simulink model "ANNC_Outer_loop_Int_Act"  (R2021b)
settings: Solver=ode4  StartTime=0.0  StopTime=35  FixedStep=1e-3  RelTol=1e-3
settings Model: Creator=hellb  LastModifiedBy=Ivan Lopez
settings SolverCC: AlgebraicLoopSolver=TrustRegion
settings DataIOCC: ReturnWorkspaceOutputs=off
settings DebuggingCC: SFMachineParentedDataDiag=warning  UnderSpecifiedDimensionMsg=warning  ArithmeticOperatorsInVariantConditions=warning
settings SFSimCC: SimUseLocalCustomCode=off  CustomCodeUndefinedFunction=UseInterfaceOnly
settings RTWCC: RTWUseLocalCustomCode=off

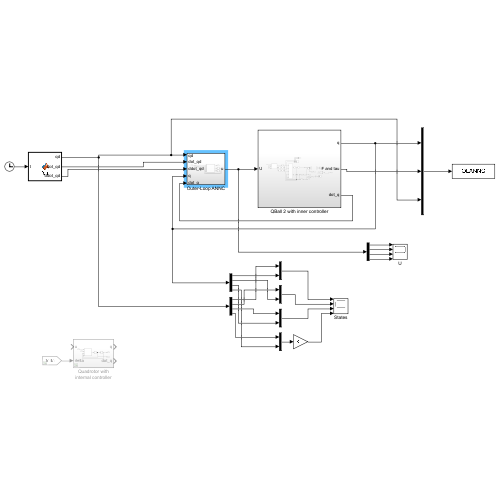
[thumbnail: Simulink's stored preview of the top-level diagram]
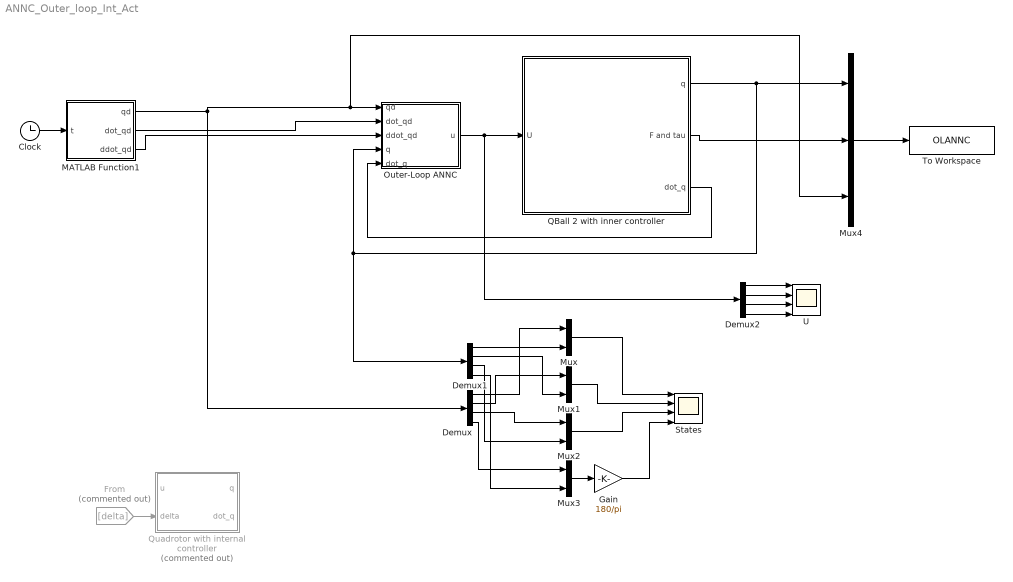
== system ANNC_Outer_loop_Int_Act ==
  Clock : Clock
  Demux : Demux
  Demux1 : Demux
  Demux2 : Demux
  From : From  Commented=on  GotoTag=delta  TagVisibility=global
  Gain : Gain  Gain=180/pi
  MATLAB Function1 : MATLAB Function  TreatAsAtomicUnit=on
  Mux{,1..3} (4 alike) : Mux  Inputs=2
  Mux4 : Mux  Inputs=3
  Outer-Loop ANNC : Subsystem
  QBall 2 with inner controller : Subsystem
  Quadrotor with internal controller : Subsystem  Commented=on
  States : Scope  NumInputPorts=4
  To Workspace : ToWorkspace  VariableName=OLANNC  SaveFormat=Structure With Time  SampleTime=-1
  U : Scope  NumInputPorts=4
  wires:
  Clock/1 -> MATLAB Function1/1(t)
  MATLAB Function1/1(qd) -> Mux4/3, Outer-Loop ANNC/1(qd), Demux/1
  Demux/1 -> Mux/1
  Demux1/1 -> Mux/2
  Demux/2 -> Mux1/1
  Demux1/2 -> Mux1/2
  Demux/3 -> Mux2/1
  Demux1/3 -> Mux2/2
  Demux/4 -> Mux3/1
  Demux1/4 -> Mux3/2
  Mux/1 -> States/1
  Mux1/1 -> States/2
  Mux2/1 -> States/3
  Mux3/1 -> Gain/1
  Gain/1 -> States/4
  From/1 -> Quadrotor with internal controller/2(delta)
  MATLAB Function1/2(dot_qd) -> Outer-Loop ANNC/2(dot_qd)
  MATLAB Function1/3(ddot_qd) -> Outer-Loop ANNC/3(ddot_qd)
  Mux4/1 -> To Workspace/1
  Outer-Loop ANNC/1(u) -> Demux2/1, QBall 2 with inner controller/1(U)
  QBall 2 with inner controller/1(q) -> Outer-Loop ANNC/4(q), Demux1/1, Mux4/1
  QBall 2 with inner controller/3(dot_q) -> Outer-Loop ANNC/5(dot_q)
  Demux2/1 -> U/1
  Demux2/2 -> U/2
  Demux2/3 -> U/3
  Demux2/4 -> U/4
  QBall 2 with inner controller/2(F and tau) -> Mux4/2

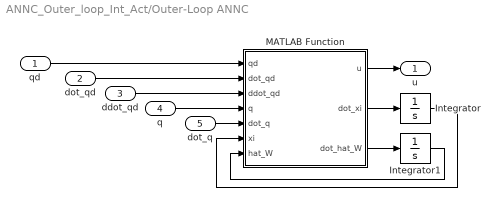
== system ANNC_Outer_loop_Int_Act/Outer-Loop ANNC ==
  qd : Inport
  dot_qd : Inport  Port=2
  ddot_qd : Inport  Port=3
  q : Inport  Port=4
  dot_q : Inport  Port=5
  Integrator : Integrator  InitialCondition=[0;0;0;0]
  Integrator1 : Integrator  InitialCondition=zeros(10,4)
  MATLAB Function : MATLAB Function  TreatAsAtomicUnit=on
  u : Outport  VectorParamsAs1DForOutWhenUnconnected=off
  wires:
  dot_q/1 -> MATLAB Function/5(dot_q)
  q/1 -> MATLAB Function/4(q)
  MATLAB Function/2(dot_xi) -> Integrator/1
  ddot_qd/1 -> MATLAB Function/3(ddot_qd)
  MATLAB Function/1(u) -> u/1
  Integrator1/1 -> MATLAB Function/7(hat_W)
  Integrator/1 -> MATLAB Function/6(xi)
  MATLAB Function/3(dot_hat_W) -> Integrator1/1
  dot_qd/1 -> MATLAB Function/2(dot_qd)
  qd/1 -> MATLAB Function/1(qd)

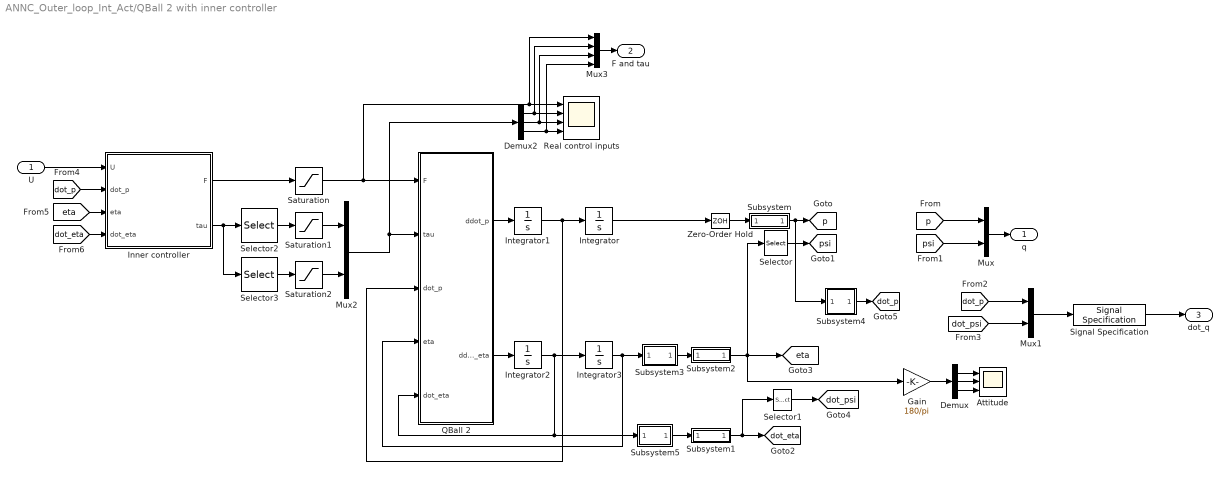
== system ANNC_Outer_loop_Int_Act/QBall 2 with inner controller ==
  U : Inport
  Attitude : Scope  NumInputPorts=3
  Demux : Demux  Outputs=3
  Demux2 : Demux  Outputs=3
  Gain : Gain  Gain=180/pi
  Inner controller : MATLAB Function  TreatAsAtomicUnit=on
  Integrator : Integrator  InitialCondition=[0;0;0.3]  LimitOutput=on  UpperSaturationLimit=[inf;inf;inf]  LowerSaturationLimit=[-inf;-inf;0.3]
  Integrator1 : Integrator  InitialCondition=[0;0;0]
  Integrator2 : Integrator  InitialCondition=[0;0;0]
  Integrator3 : Integrator  InitialCondition=[0;0;0]  LimitOutput=on  UpperSaturationLimit=[pi/2; pi/2; inf]  LowerSaturationLimit=[-pi/2; -pi/2; -inf]
  Mux : Mux  Inputs=2
  Mux1 : Mux  Inputs=2
  Mux2 : Mux  Inputs=2
  Mux3 : Mux
  QBall 2 : MATLAB Function  TreatAsAtomicUnit=on
  Real control inputs : Scope  NumInputPorts=4
  Saturation : Saturate  UpperLimit=8.6*4  LowerLimit=0
  Saturation1 : Saturate  UpperLimit=0.7  LowerLimit=-0.7
  Saturation2 : Saturate  UpperLimit=0.43  LowerLimit=-0.43
  Selector : Selector  InputPortWidth=3  IndexOptions=Index vector (dialog)  Indices=[3]  OutputSizes=1
  Selector1 : Selector  InputPortWidth=3  IndexOptions=Index vector (dialog)  Indices=[3]  OutputSizes=1
  Selector2 : Selector  InputPortWidth=3  IndexOptions=Index vector (dialog)  Indices=[1 2]  OutputSizes=1
  Selector3 : Selector  InputPortWidth=3  IndexOptions=Index vector (dialog)  Indices=[3]  OutputSizes=1
  Signal Specification : SignalSpecification  Dimensions=4
  Subsystem : Subsystem
  Subsystem1 : Subsystem
  Subsystem2 : Subsystem
  Subsystem3 : Subsystem
  Subsystem4 : Subsystem
  Subsystem5 : Subsystem
  Zero-Order Hold : ZeroOrderHold  SampleTime=0.033
  q : Outport
  F and tau : Outport  Port=2
  dot_q : Outport  Port=3
  tag scope: dot_eta=global, dot_p=global, dot_psi=global, eta=global, p=global, psi=global
  wires:
  Integrator3/1 -> Subsystem3/1(In1), QBall 2/4(eta)
  QBall 2/2(ddot_eta) -> Integrator2/1
  QBall 2/1(ddot_p) -> Integrator1/1
  Integrator2/1 -> Subsystem5/1(In1), QBall 2/5(dot_eta), Integrator3/1
  Integrator/1 -> Zero-Order Hold/1
  Mux/1 -> q/1
  Integrator1/1 -> QBall 2/3(dot_p), Integrator/1
  Inner controller/1(F) -> Saturation/1
  Inner controller/2(tau) -> Selector3/1, Selector2/1
  Selector2/1 -> Saturation1/1
  Selector3/1 -> Saturation2/1
  Saturation1/1 -> Mux2/1
  Saturation2/1 -> Mux2/2
  U/1 -> Inner controller/1(U)
  Saturation/1 -> Mux3/1, Real control inputs/1, QBall 2/1(F)
  Mux2/1 -> Demux2/1, QBall 2/2(tau)
  Demux/1 -> Attitude/1
  Demux/2 -> Attitude/2
  Demux/3 -> Attitude/3
  Demux2/1 -> Mux3/2, Real control inputs/2
  Demux2/2 -> Mux3/3, Real control inputs/3
  Demux2/3 -> Mux3/4, Real control inputs/4
  Gain/1 -> Demux/1
  Mux3/1 -> F and tau/1
  Zero-Order Hold/1 -> Subsystem/1(In1)
  Subsystem/1(Out1) -> Subsystem4/1(In1), [p]
  Subsystem1/1(Out1) -> Selector1/1, [dot_eta]
  Subsystem2/1(Out1) -> Gain/1, Selector/1, [eta]
  Subsystem3/1(Out1) -> Subsystem2/1(In1)
  Selector/1 -> [psi]
  Selector1/1 -> [dot_psi]
  Subsystem4/1(Out1) -> [dot_p]
  [p] -> Mux/1
  [psi] -> Mux/2
  [dot_p] -> Inner controller/2(dot_p)
  [eta] -> Inner controller/3(eta)
  [dot_eta] -> Inner controller/4(dot_eta)
  [dot_psi] -> Mux1/2
  [dot_p] -> Mux1/1
  Mux1/1 -> Signal Specification/1
  Signal Specification/1 -> dot_q/1
  Subsystem5/1(Out1) -> Subsystem1/1(In1)

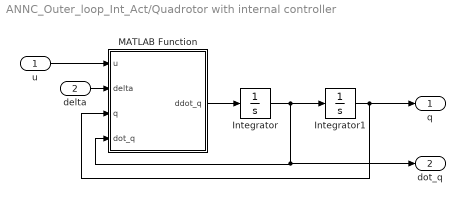
== system ANNC_Outer_loop_Int_Act/Quadrotor with internal controller ==
  u : Inport
  delta : Inport  Port=2
  Integrator : Integrator  InitialCondition=[0;0;0;0]
  Integrator1 : Integrator  InitialCondition=[0;0;0.3;deg2rad(2)]
  MATLAB Function : MATLAB Function  TreatAsAtomicUnit=on
  q : Outport  VectorParamsAs1DForOutWhenUnconnected=off
  dot_q : Outport  Port=2  VectorParamsAs1DForOutWhenUnconnected=off
  wires:
  Integrator/1 -> dot_q/1, MATLAB Function/4(dot_q), Integrator1/1
  Integrator1/1 -> q/1, MATLAB Function/3(q)
  MATLAB Function/1(ddot_q) -> Integrator/1
  u/1 -> MATLAB Function/1(u)
  delta/1 -> MATLAB Function/2(delta)

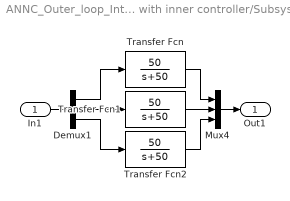
== system ANNC_Outer_loop_Int_Act/QBall 2 with inner controller/Subsystem ==
  In1 : Inport
  Demux1 : Demux  Outputs=3
  Mux4 : Mux  Inputs=3
  Transfer Fcn : TransferFcn  Numerator=[50]  Denominator=[1 50]
  Transfer Fcn1 : TransferFcn  Numerator=[50]  Denominator=[1 50]
  Transfer Fcn2 : TransferFcn  Numerator=[50]  Denominator=[1 50]
  Out1 : Outport
  wires:
  Transfer Fcn2/1 -> Mux4/3
  Mux4/1 -> Out1/1
  Transfer Fcn/1 -> Mux4/1
  Transfer Fcn1/1 -> Mux4/2
  Demux1/2 -> Transfer Fcn1/1
  Demux1/3 -> Transfer Fcn2/1
  Demux1/1 -> Transfer Fcn/1
  In1/1 -> Demux1/1

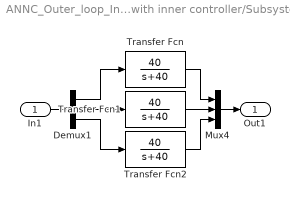
== system ANNC_Outer_loop_Int_Act/QBall 2 with inner controller/Subsystem1 ==
  In1 : Inport
  Demux1 : Demux  Outputs=3
  Mux4 : Mux  Inputs=3
  Transfer Fcn : TransferFcn  Numerator=[40]  Denominator=[1 40]
  Transfer Fcn1 : TransferFcn  Numerator=[40]  Denominator=[1 40]
  Transfer Fcn2 : TransferFcn  Numerator=[40]  Denominator=[1 40]
  Out1 : Outport
  wires:
  In1/1 -> Demux1/1
  Demux1/1 -> Transfer Fcn/1
  Demux1/3 -> Transfer Fcn2/1
  Demux1/2 -> Transfer Fcn1/1
  Transfer Fcn1/1 -> Mux4/2
  Transfer Fcn/1 -> Mux4/1
  Mux4/1 -> Out1/1
  Transfer Fcn2/1 -> Mux4/3

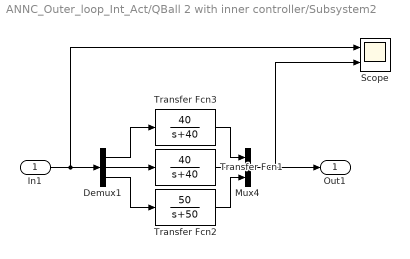
== system ANNC_Outer_loop_Int_Act/QBall 2 with inner controller/Subsystem2 ==
  In1 : Inport
  Demux1 : Demux  Outputs=3
  Mux4 : Mux  Inputs=3
  Scope : Scope  NumInputPorts=2
  Transfer Fcn1 : TransferFcn  Numerator=[40]  Denominator=[1 40]
  Transfer Fcn2 : TransferFcn  Numerator=[50]  Denominator=[1 50]
  Transfer Fcn3 : TransferFcn  Numerator=[40]  Denominator=[1 40]
  Out1 : Outport
  wires:
  Transfer Fcn2/1 -> Mux4/3
  Mux4/1 -> Scope/2, Out1/1
  Transfer Fcn3/1 -> Mux4/1
  Transfer Fcn1/1 -> Mux4/2
  Demux1/2 -> Transfer Fcn1/1
  Demux1/3 -> Transfer Fcn2/1
  Demux1/1 -> Transfer Fcn3/1
  In1/1 -> Scope/1, Demux1/1

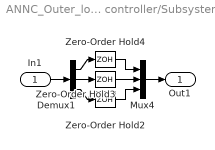
== system ANNC_Outer_loop_Int_Act/QBall 2 with inner controller/Subsystem3 ==
  In1 : Inport
  Demux1 : Demux  Outputs=3
  Mux4 : Mux  Inputs=3
  Zero-Order Hold2 : ZeroOrderHold  SampleTime=0.033
  Zero-Order Hold3 : ZeroOrderHold  SampleTime=0.002
  Zero-Order Hold4 : ZeroOrderHold  SampleTime=0.002
  Out1 : Outport
  wires:
  Zero-Order Hold4/1 -> Mux4/1
  In1/1 -> Demux1/1
  Zero-Order Hold2/1 -> Mux4/3
  Demux1/3 -> Zero-Order Hold2/1
  Zero-Order Hold3/1 -> Mux4/2
  Demux1/2 -> Zero-Order Hold3/1
  Demux1/1 -> Zero-Order Hold4/1
  Mux4/1 -> Out1/1

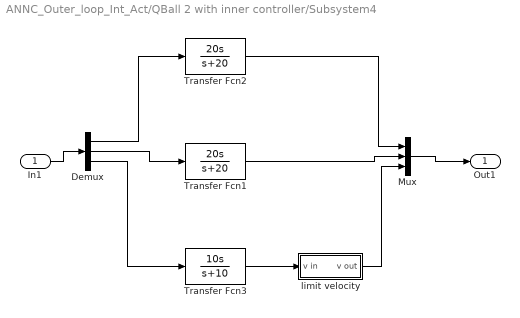
== system ANNC_Outer_loop_Int_Act/QBall 2 with inner controller/Subsystem4 ==
  In1 : Inport
  Demux : Demux  Outputs=3
  Mux : Mux  Inputs=3
  Transfer Fcn1 : TransferFcn  Numerator=[20 0]  Denominator=[1 20]
  Transfer Fcn2 : TransferFcn  Numerator=[20 0]  Denominator=[1 20]
  Transfer Fcn3 : TransferFcn  Numerator=[10 0]  Denominator=[1 10]
  limit velocity : Subsystem
  Out1 : Outport
  wires:
  Transfer Fcn3/1 -> limit velocity/1(v in)
  limit velocity/1(v out) -> Mux/3
  Transfer Fcn1/1 -> Mux/2
  Transfer Fcn2/1 -> Mux/1
  Demux/2 -> Transfer Fcn1/1
  Demux/1 -> Transfer Fcn2/1
  Demux/3 -> Transfer Fcn3/1
  In1/1 -> Demux/1
  Mux/1 -> Out1/1

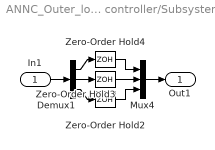
== system ANNC_Outer_loop_Int_Act/QBall 2 with inner controller/Subsystem5 ==
  In1 : Inport
  Demux1 : Demux  Outputs=3
  Mux4 : Mux  Inputs=3
  Zero-Order Hold2 : ZeroOrderHold  SampleTime=0.002
  Zero-Order Hold3 : ZeroOrderHold  SampleTime=0.002
  Zero-Order Hold4 : ZeroOrderHold  SampleTime=0.002
  Out1 : Outport
  wires:
  Mux4/1 -> Out1/1
  Demux1/1 -> Zero-Order Hold4/1
  Demux1/2 -> Zero-Order Hold3/1
  Zero-Order Hold3/1 -> Mux4/2
  Demux1/3 -> Zero-Order Hold2/1
  Zero-Order Hold2/1 -> Mux4/3
  In1/1 -> Demux1/1
  Zero-Order Hold4/1 -> Mux4/1

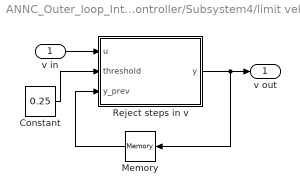
== system ANNC_Outer_loop_Int_Act/QBall 2 with inner controller/Subsystem4/limit velocity ==
  v in : Inport
  Constant : Constant  Value=0.25
  Memory : Memory  InheritSampleTime=on
  Reject steps in v : MATLAB Function  TreatAsAtomicUnit=on
  v out : Outport
  wires:
  Reject steps in v/1(y) -> Memory/1, v out/1
  Constant/1 -> Reject steps in v/2(threshold)
  Memory/1 -> Reject steps in v/3(y_prev)
  v in/1 -> Reject steps in v/1(u)

== matlab function ANNC_Outer_loop_Int_Act/Outer-Loop ANNC/MATLAB Function ==
  settings: updateMethod=DISCRETE
  data: qd input; u output; dot_qd input; ddot_qd input; q input; dot_q input; xi input; dot_xi output; dot_hat_W output; hat_W input
function [u, dot_xi, dot_hat_W] = fcn(qd, dot_qd, ddot_qd, q, dot_q, xi, hat_W)

% Controller parameters
fm = 0.3;
Kp = fm*diag([0.5 0.5 0.8 0.5]);
Kd = fm*diag([0.5 0.5 0.5 0.5]);
Ki = 1*diag([0.001 0.001 0.001 0.001]);
Delta = 0.001*diag([1 1 1 1]);
alpha = 0.33;
% %%%%%%%%%%%%%%%%%%%%%
psi    = q(4);
e      = qd - q;
dot_e  = dot_qd - dot_q;
dot_xi = alpha*e + dot_e;
gamma  = [1; ddot_qd; dot_q];

% ANN parameters
LN = 10; % Quantity of neurons
rng(0,'twister'); % Initialization of the random number genrerator to make the values repitable
V = 2.*rand(length(gamma),LN) - 1; % Matrix with values in [-1, 1]
N = 0.005*diag(LN);
k = 0.001;
% %%%%%%%%%%%%%%
sigma = tanh(V'*gamma);
dot_hat_W = N*(sigma*dot_xi' - k*norm(dot_xi)*hat_W);

T  = [cos(psi)  sin(psi) 0 0
      sin(psi) -cos(psi) 0 0
      0         0        1 0
      0         0        0 1];

u = T\(Kp*e + Ki*xi + Kd*dot_e + 1*hat_W'*sigma + Delta*sign(dot_xi));

== matlab function ANNC_Outer_loop_Int_Act/Quadrotor with internal controller/MATLAB Function ==
  data: u input; ddot_q output; delta input; q input; dot_q input
function ddot_q = fcn(u, delta, q, dot_q)
psi = q(4);
% Parametros tomados del articulo de Adaptive GRNNC
% correspondientes al QBall 2 de Quanser.
g = 9.81;
m = 1.79;
tht_max = deg2rad(92.35);
phi_max = deg2rad(92.35);
dotz_max = 7.7168;
dotpsi_max = deg2rad(99.2730);
tau_dotz   = 0.728;
tau_dotpsi = 0.728;
dx = 0.2;
dy = 0.2;
dz = 0.4;
% %%%%%%%%%%%%%%%%%%%%%%%%%%%%%%%%%%%%%%%%%%%%%%%%%
Ku = diag([g*tht_max g*phi_max dotz_max/tau_dotz dotpsi_max/tau_dotpsi]);
Kv = diag([dx dy ((1/tau_dotz)+(dz/m)) 1/tau_dotpsi]);

T  = [cos(psi)  sin(psi) 0 0
      sin(psi) -cos(psi) 0 0
      0         0        1 0
      0         0        0 1];
  
ddot_q = T*Ku*u - Kv*dot_q + delta;

== matlab function ANNC_Outer_loop_Int_Act/MATLAB Function1 ==
  data: t input; qd output; dot_qd output; ddot_qd output
function [qd, dot_qd, ddot_qd] = fcn(t)

xfreq = 2*pi/4;
yfreq = 2*pi/8;
xamp = 0.5;
yamp = 1;
hf = 1;
h0 = 0.3;
b = 0.1;

if t <= 5
qd = [xamp*sin(xfreq*t)
      yamp*cos(yfreq*t)
      hf - exp(-b*t^3)*(hf - h0)
      0];

dot_qd = [xfreq*xamp*cos(xfreq*t)
          -yfreq*yamp*sin(yfreq*t)
          3*b*t^2*exp(-b*t^3)*(hf - h0)
          0];
ddot_qd = [-xfreq^2*xamp*sin(xfreq*t)
           -yfreq^2*yamp*cos(yfreq*t)
           6*b*t*exp(-b*t^3)*(hf - h0) - 9*b^2*t^4*exp(-b*t^3)*(hf - h0)
           0];
else
    qd = [xamp*sin(xfreq*t)
      yamp*cos(yfreq*t)
      1
      0];

dot_qd = [xfreq*xamp*cos(xfreq*t)
          -yfreq*yamp*sin(yfreq*t)
          0
          0];
ddot_qd = [-xfreq^2*xamp*sin(xfreq*t)
           -yfreq^2*yamp*cos(yfreq*t)
           0
           0];
end

== matlab function ANNC_Outer_loop_Int_Act/QBall 2 with inner controller/QBall 2 ==
  data: F input; tau input; ddot_p output; ddot_eta output; dot_p input; eta input; dot_eta input
function [ddot_p, ddot_eta] = fcn(F, tau, dot_p, eta, dot_eta)

m  = 1.79;
g  = 9.81;

Ixx = 0.03; Iyy = 0.03; Izz = 0.04;
dx = 0.002; dy = 0.002; dz = 0.004;
d_phi = 0.002; d_theta = 0.002; d_psi = 0.004;
I  = diag([Ixx Iyy Izz]);
Dp = diag([dx dy dz]);
Dn = diag([d_phi d_theta d_psi]);
Vz = [0; 0; 1];

phi     = eta(1);     theta     = eta(2);     psi = eta(3);
dot_phi = dot_eta(1); dot_theta = dot_eta(2);

R = [cos(theta)*cos(psi)  sin(phi)*sin(theta)*cos(psi)-cos(phi)*sin(psi)  cos(phi)*sin(theta)*cos(psi)+sin(phi)*sin(psi)
     cos(theta)*sin(psi)  sin(phi)*sin(theta)*sin(psi)+cos(phi)*cos(psi)  cos(phi)*sin(theta)*sin(psi)-sin(phi)*cos(psi)
     -sin(theta)          sin(phi)*cos(theta)                             cos(phi)*cos(theta)];
 
% W = [1  sin(phi)*tan(theta)  cos(phi)*tan(theta)
%      0  cos(phi)             -sin(phi)
%      0  sin(phi)/cos(theta)  cos(phi)/cos(theta)];

iW = [1 0         -sin(theta)
      0 cos(phi)  cos(theta)*sin(phi)
      0 -sin(phi) cos(theta)*cos(phi)];
 
dot_W = [0  (cos(phi)*tan(theta))+((sin(phi)*dot_theta)/(cos(theta)^2))                     ((cos(phi)*dot_theta)/(cos(theta)^2))-(sin(phi)*tan(theta)*dot_phi)
         0  -sin(phi)*dot_phi                                                               -cos(phi)*dot_phi
         0  ((cos(phi)*cos(theta)*dot_phi)+(sin(phi)*sin(theta)*dot_theta))/(cos(theta)^2)  ((cos(phi)*sin(theta)*dot_theta)-(sin(phi)*cos(theta)*dot_phi))/(cos(theta)^2)];
  
iWdot_eta = iW*dot_eta;

SiWdot_eta = [0              -iWdot_eta(3)  iWdot_eta(2)
              iWdot_eta(3)   0              -iWdot_eta(1)
              -iWdot_eta(2)  iWdot_eta(1)   0];

M = iW'*I*iW;
C = iW'*(SiWdot_eta*I - I*iW*dot_W)*iW;
l = 0.2;
kv = 0.5;
B = [1 1 1 1; 0 -l 0 l; -l 0 l 0; -kv kv -kv kv];
Gamma = diag([0 0 0 0]);
u = [F; tau(1); tau(2); tau(3)];

u_bar = B*((eye(4)-Gamma)*(B\u));
F_bar = u_bar(1);
tau_bar = [u_bar(2); u_bar(3); u_bar(4)];

ddot_p   = (R*Vz*F_bar - m*g*Vz - Dp*dot_p)/m;
ddot_eta = M\(iW'*tau_bar - C*dot_eta - Dn*dot_eta);

== matlab function ANNC_Outer_loop_Int_Act/QBall 2 with inner controller/Inner controller ==
  data: U input; F output; tau output; dot_p input; eta input; dot_eta input
function [F, tau] = fcn(U, dot_p, eta, dot_eta)

m  = 1.79;
g  = 9.81;

dot_zmax   = 7.7168;
phi_max    = 1.6118;
theta_max  = phi_max;
dot_psimax = dot_zmax;

omega_phi   = 13.994;
omega_theta = omega_phi;
xi_phi      = 1.593;
xi_theta    = xi_phi;
tau_dotz    = 0.728;
tau_dotpsi  = tau_dotz;

Ixx = 0.03; Iyy = 0.03; Izz = 0.04;
I  = diag([Ixx Iyy Izz]);

dot_z   = dot_p(3);
phi     = eta(1);     theta     = eta(2);
dot_phi = dot_eta(1); dot_theta = dot_eta(2); dot_psi = dot_eta(3);
 
W = [1  sin(phi)*tan(theta)  cos(phi)*tan(theta)
     0  cos(phi)             -sin(phi)
     0  sin(phi)/cos(theta)  cos(phi)/cos(theta)];

iW = [1 0         -sin(theta)
      0 cos(phi)  cos(theta)*sin(phi)
      0 -sin(phi) cos(theta)*cos(phi)];
 
dot_W = [0  (cos(phi)*tan(theta))+((sin(phi)*dot_theta)/(cos(theta)^2))                     ((cos(phi)*dot_theta)/(cos(theta)^2))-(sin(phi)*tan(theta)*dot_phi)
         0  -sin(phi)*dot_phi                                                               -cos(phi)*dot_phi
         0  ((cos(phi)*cos(theta)*dot_phi)+(sin(phi)*sin(theta)*dot_theta))/(cos(theta)^2)  ((cos(phi)*sin(theta)*dot_theta)-(sin(phi)*cos(theta)*dot_phi))/(cos(theta)^2)];
  
iWdot_eta = iW*dot_eta;

SiWdot_eta = [0              -iWdot_eta(3)  iWdot_eta(2)
              iWdot_eta(3)   0              -iWdot_eta(1)
              -iWdot_eta(2)  iWdot_eta(1)   0];

M = iW'*I*iW;
C = iW'*(SiWdot_eta*I - I*iW*dot_W)*iW;


theta_d  = theta_max*U(1);
phi_d    = phi_max*U(2);
dot_zd   = dot_zmax*U(3);
dot_psid = dot_psimax*U(4);

dot_zstar = (dot_zd - dot_z)/tau_dotz;
tau_tilde = [omega_phi^2*(phi_d - phi) - 2*xi_phi*omega_phi*dot_phi
             omega_theta^2*(theta_d - theta) - 2*xi_theta*omega_theta*dot_theta
             (dot_psid - dot_psi)/tau_dotpsi];

F   = (m*(g + dot_zstar))/(cos(phi)*cos(theta));
tau = W'*(M*tau_tilde + C*dot_eta);

== matlab function ANNC_Outer_loop_Int_Act/QBall 2 with inner controller/Subsystem4/limit velocity/Reject steps in v ==
  data: u input; y output; threshold input; y_prev input
function y = fcn(u, threshold, y_prev)
% This block supports the Embedded MATLAB subset.
% See the help menu for details. 

if abs(u - y_prev) > threshold
    y = y_prev;
else
    y = u;
end
